simulink model "Heating_System_Simulink"  (R2022a)
settings: Solver=VariableStepAuto  StartTime=0.0  StopTime=10  FixedStep=0.05  RelTol=1e-3
model workspace (MAT data in the model file):
  M = 4.375
  Mdot = 10
  Req = 0.001
  c = 1005
libraries: slpidlib x1
settings Model: Creator=vamsi  LastModifiedBy=vamsi

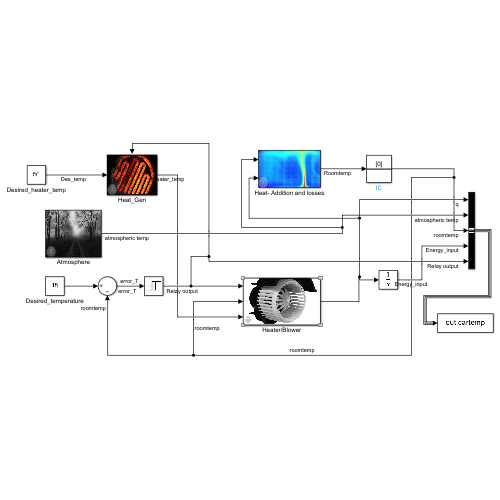
[thumbnail: Simulink's stored preview of the top-level diagram]
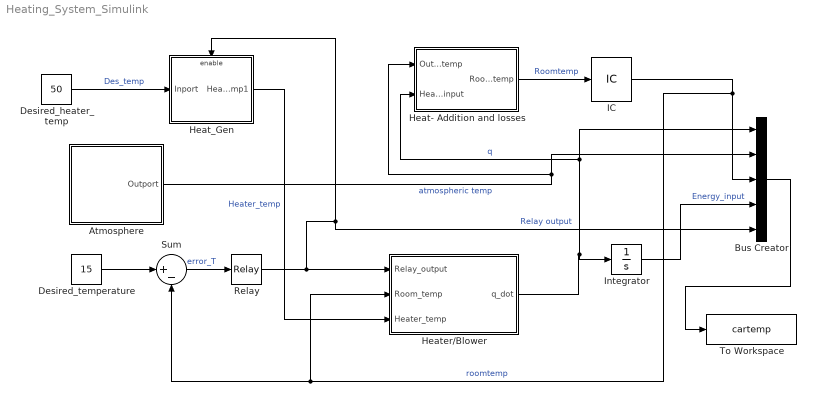
== system Heating_System_Simulink ==
  Atmosphere : Subsystem
      mask Display: image('atm.jpg');
  Bus Creator : BusCreator  Inputs=5
  Desired_heater_temp : Constant  Value=50
  Desired_temperature : Constant  Value=15
  Heat- Addition and losses : Subsystem
      mask Display: image('heat4.png')
  Heat_Gen : Subsystem  TreatAsAtomicUnit=on
      mask Display: image('coil.jpg');
  Heater/Blower : Subsystem
      mask Display: image('blower.jpg')
  IC : InitialCondition  Value=0
  Integrator : Integrator
  Relay : Relay  OnSwitchValue=1  OffSwitchValue=-1
  Sum : Sum  Inputs=|+-
  To Workspace : ToWorkspace  VariableName=cartemp  SaveFormat=Timeseries  SampleTime=-1
  wires:
  Desired_temperature/1 -> Sum/1
  Sum/1 -> Relay/1  "error_T"
  Heat- Addition and losses/1(Room_temp) -> IC/1  "Roomtemp"
  Heater/Blower/1(q_dot) -> Heat- Addition and losses/2(Heat_input), Bus Creator/1, Integrator/1  "q"
  Atmosphere/1(Outport) -> Heat- Addition and losses/1(Outside_temp), Bus Creator/2  "atmospheric temp"
  Heat_Gen/1(Heater_temp1) -> Heater/Blower/3(Heater_temp)  "Heater_temp"
  Desired_heater_temp/1 -> Heat_Gen/1(Inport)  "Des_temp"
  Integrator/1 -> Bus Creator/4  "Energy_input"
  Bus Creator/1 -> To Workspace/1
  IC/1 -> Sum/2, Heater/Blower/2(Room_temp), Bus Creator/3  "roomtemp"
  Relay/1 -> Bus Creator/5, Heat_Gen/Enable, Heater/Blower/1(Relay_output)  "Relay output"

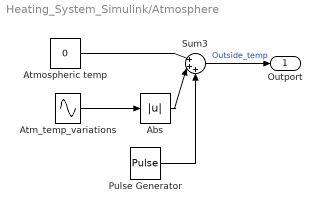
== system Heating_System_Simulink/Atmosphere ==
  Abs : Abs  SaturateOnIntegerOverflow=off
  Atm_temp_variations : Sin  Amplitude=2  Frequency=pi/10  SampleTime=0
  Atmospheric temp : Constant  Value=0
  Pulse Generator : DiscretePulseGenerator  PulseType=Time based  Amplitude=0.8  Period=10  PulseWidth=30  PhaseDelay=4
  Sum3 : Sum  Inputs=|+++
  Outport : Outport
  wires:
  Atm_temp_variations/1 -> Abs/1
  Sum3/1 -> Outport/1  "Outside_temp"
  Atmospheric temp/1 -> Sum3/1
  Abs/1 -> Sum3/2
  Pulse Generator/1 -> Sum3/3

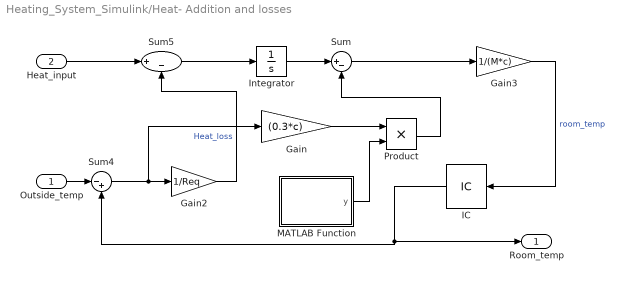
== system Heating_System_Simulink/Heat- Addition and losses ==
  Outside_temp : Inport
  Heat_input : Inport  Port=2
  Gain : Gain  Gain=(0.3*c)
  Gain2 : Gain  Gain=1/Req
  Gain3 : Gain  Gain=1/(M*c)
  IC : InitialCondition  Value=0
  Integrator : Integrator  InitialCondition=30
  MATLAB Function : MATLAB Function  TreatAsAtomicUnit=on
  Product : Product
  Sum : Sum  Inputs=|+-
  Sum4 : Sum  Inputs=|-+
  Sum5 : Sum  Inputs=|+-
  Room_temp : Outport
  wires:
  Gain2/1 -> Sum5/2  "Heat_loss"
  Outside_temp/1 -> Sum4/1
  Heat_input/1 -> Sum5/1
  MATLAB Function/1(y) -> Product/2
  Gain/1 -> Product/1
  Gain3/1 -> IC/1  "room_temp"
  Product/1 -> Sum/2
  IC/1 -> Sum4/2, Room_temp/1
  Sum4/1 -> Gain/1, Gain2/1
  Sum/1 -> Gain3/1
  Integrator/1 -> Sum/1
  Sum5/1 -> Integrator/1

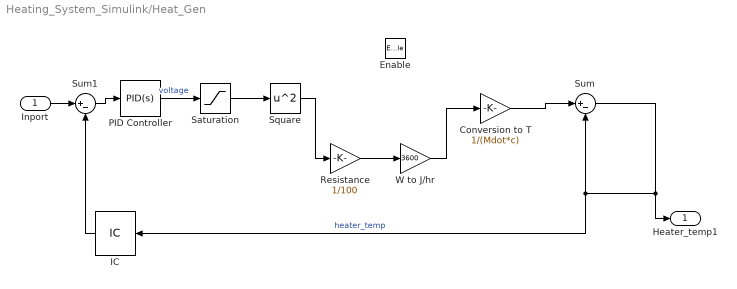
== system Heating_System_Simulink/Heat_Gen ==
  Inport : Inport
  Enable : EnablePort  StatesWhenEnabling=reset
  Conversion to T : Gain  Gain=1/(Mdot*c)
  IC : InitialCondition  Value=0
  PID Controller : slpidlib/PID Controller  Controller=PID  Form=Parallel  TimeDomain=Continuous-time  UseExternalTs=off  SampleTime=-1  IntegratorMethod=Forward Euler  FilterMethod=Forward Euler  ControllerParametersSource=internal  P=5000  I=1  UseKiTs=off  D=0  N=150  UseFilter=on  TunerSelectOption=Transfer Function Based (PID Tuner App)  InitialConditionSource=internal  InitialConditionForIntegrator=0  InitialConditionForFilter=0  DifferentiatorICPrevScaledInput=0  ExternalReset=none  TrackingMode=off  Kt=1  LimitOutput=off  SatLimitsSource=internal  UpperSaturationLimit=inf  LowerSaturationLimit=-inf  LinearizeAsGain=on  AntiWindupMode=none  Kb=1  POutMin=[]  POutMax=[]  IOutMin=[]  IOutMax=[]  DOutMin=[]  DOutMax=[]  NOutMin=[]  NOutMax=[]  SumOutMin=[]  SumOutMax=[]  SaturationOutMin=[]  SaturationOutMax=[]  PParamMin=[]  PParamMax=[]  IParamMin=[]  IParamMax=[]  DParamMin=[]  DParamMax=[]  NParamMin=[]  NParamMax=[]  KbParamMin=[]  KbParamMax=[]  KtParamMin=[]  KtParamMax=[]  KbOutMin=[]  KbOutMax=[]  KtOutMin=[]  KtOutMax=[]  IntegratorOutMin=[]  IntegratorOutMax=[]  FilterOutMin=[]  FilterOutMax=[]  SumI1OutMin=[]  SumI1OutMax=[]  SumI2OutMin=[]  SumI2OutMax=[]  SumI3OutMin=[]  SumI3OutMax=[]  SumI4OutMin=[]  SumI4OutMax=[]  SumDOutMin=[]  SumDOutMax=[]  DifferentiatorOutMin=[]  DifferentiatorOutMax=[]  FilterDiffOutCoefMin=[]  FilterDiffOutCoefMax=[]  ReciprocalOutMin=[]  ReciprocalOutMax=[]  SumDenOutMin=[]  SumDenOutMax=[]  SumNumOutMin=[]  SumNumOutMax=[]  DivideOutMin=[]  DivideOutMax=[]  UdiffTsProdOutMin=[]  UdiffTsProdOutMax=[]  NTsProdOutMin=[]  NTsProdOutMax=[]  UintegralTsProdOutMin=[]  UintegralTsProdOutMax=[]  UngainTsProdOutMin=[]  UngainTsProdOutMax=[]  IntegratorContinuousStateAttributes=''  IntegratorStateMustResolveToSignalObject=off  IntegratorRTWStateStorageClass=Auto  FilterContinuousStateAttributes=''  FilterStateMustResolveToSignalObject=off  FilterRTWStateStorageClass=Auto  ParallelPVariant=InternalParameters  IdealPVariant=Disabled  IVariant=InternalParameters  DVariant=InternalParameters  IntegratorVariant=Continuous  SatVariant=Disabled  AWVariant=Passthrough  PCopyVariant=Disabled  TRVariant=Disabled  FdbkBlocksVariant=Forward  IdealPFdbkVariant=Disabled  SatFdbkVariant=Disabled  DerivativeFilterVariant=ContFilter  NVariant=InternalParameters  NCopyVariant=Disabled  FilterICVariant=InternalICsFilter  IntegratorICVariant=InternalICs  ExternalResetVariant=Disabled  TRSumVariant=Passthrough  SumFdbkVariant=Disabled  SumVariant=Sum_PID  TsampFilterVariant=InternalTs  TsampNgainVariant=Passthrough  TsampIntegralVariant=Passthrough  ExternalSaturationOutDataTypeStr=Inherit: Same as second input  aMode=0
  Resistance : Gain  Gain=1/100
      mask Display: image("resistance.png")
  Saturation : Saturate  UpperLimit=220  LowerLimit=0
  Square : Math  Operator=square
  Sum : Sum  Inputs=|+-
  Sum1 : Sum  Inputs=|+-
  W to J/hr : Gain  Gain=3600
  Heater_temp1 : Outport
  wires:
  Sum/1 -> Heater_temp1/1, IC/1, Sum/2  "heater_temp"
  Conversion to T/1 -> Sum/1
  Square/1 -> Resistance/1
  IC/1 -> Sum1/2
  Inport/1 -> Sum1/1
  Sum1/1 -> PID Controller/1
  W to J/hr/1 -> Conversion to T/1
  Resistance/1 -> W to J/hr/1
  Saturation/1 -> Square/1
  PID Controller/1 -> Saturation/1  "voltage"

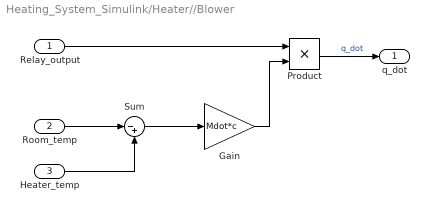
== system Heating_System_Simulink/Heater//Blower ==
  Relay_output : Inport
  Room_temp : Inport  Port=2
  Heater_temp : Inport  Port=3
  Gain : Gain  Gain=Mdot*c
  Product : Product
  Sum : Sum  Inputs=|-+
  q_dot : Outport
  wires:
  Product/1 -> q_dot/1  "q_dot"
  Room_temp/1 -> Sum/1
  Heater_temp/1 -> Sum/2
  Relay_output/1 -> Product/1
  Sum/1 -> Gain/1
  Gain/1 -> Product/2

== matlab function Heating_System_Simulink/Heat- Addition and losses/MATLAB Function ==
  data: y output
function y = window()

y = rand(1,1);
